simulink model "PWMcode1"  (R2017b)
settings: Solver=VariableStepAuto  StartTime=0.0  StopTime=10.0  RelTol=1e-3
settings Model: Creator=Gali  LastModifiedBy=Gali

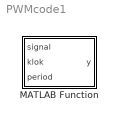
== system PWMcode1 ==
  MATLAB Function : MATLAB Function  TreatAsAtomicUnit=on

== matlab function PWMcode1/MATLAB Function ==
  data: signal input; y output; klok input; period input
function y = fcn(signal, klok, period)

    %#codegen

    minValue=0.0;

    maxValue=100.0;

    duty=(signal-minValue)/(maxValue-minValue);

    intvalue=floor(klok/period);

    cduty=klok/period-intvalue;

    if cduty<duty

        y=1;

    else

        y=0;

    end
